simulink model "simulation_lab6"  (R2022b)
settings: Solver=FixedStepAuto  StartTime=0.0  StopTime=30  FixedStep=0.001  RelTol=1e-3
values from neighbouring files (symbols this model uses):
  A = double(subs(A,par,value))    [Lab6.m]    (also in Lab6_shu.m = [0  1                                                       )
  B = double(subs(B,par,value))    [Lab6.m]    (also in Lab6_shu.m = [0)
  C = [1 0 0 0;0 0 1 0]    [Lab6.m]    (also in Lab6_shu.m = [C1; C2])
  Cy = [1 0 0 0]    [Lab6.m]    (also in Lab6_shu.m)
  Cy_theta = [1 0 0 0;0 0 1 0]    [Lab6.m]    (also in Lab6_shu.m = [1 0 0 0; 0 0 1 0])
  D = zeros(2,1)    [Lab6.m]    (also in Lab6_shu.m = [0])
  Ly_fast = place(A',180/pi*Cy',poles_modified*6)'    [Lab6.m]    (also in Lab6_shu.m = (place(A',180/pi*Cy',6*poles))')
  Ly_slow = place(A',180/pi*Cy',poles_modified*3)'    [Lab6.m]    (also in Lab6_shu.m = (place(A',180/pi*Cy',3*poles))')
  Ly_theta_fast = place(A',180/pi*Cy_theta',poles_modified*6)'    [Lab6.m]    (also in Lab6_shu.m = (place(A',180/pi*Cy_theta',6*poles))')
  Ly_theta_slow = place(A',180/pi*Cy_theta',poles_modified*3)'    [Lab6.m]    (also in Lab6_shu.m = (place(A',180/pi*Cy_theta',3*poles))')
settings Model: Creator=me-clab2  LastModifiedBy=X1
settings SolverCC: AlgebraicLoopSolver=TrustRegion
settings DebuggingCC: UnconnectedInputMsg=warning  UnconnectedOutputMsg=warning  UnconnectedLineMsg=warning  SFMachineParentedDataDiag=warning
settings ModelReferenceCC: EnableRefExpFcnMdlSchedulingChecks=on

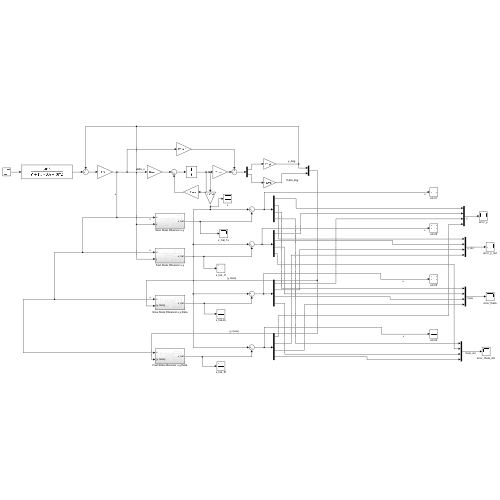
[thumbnail: Simulink's stored preview of the top-level diagram]
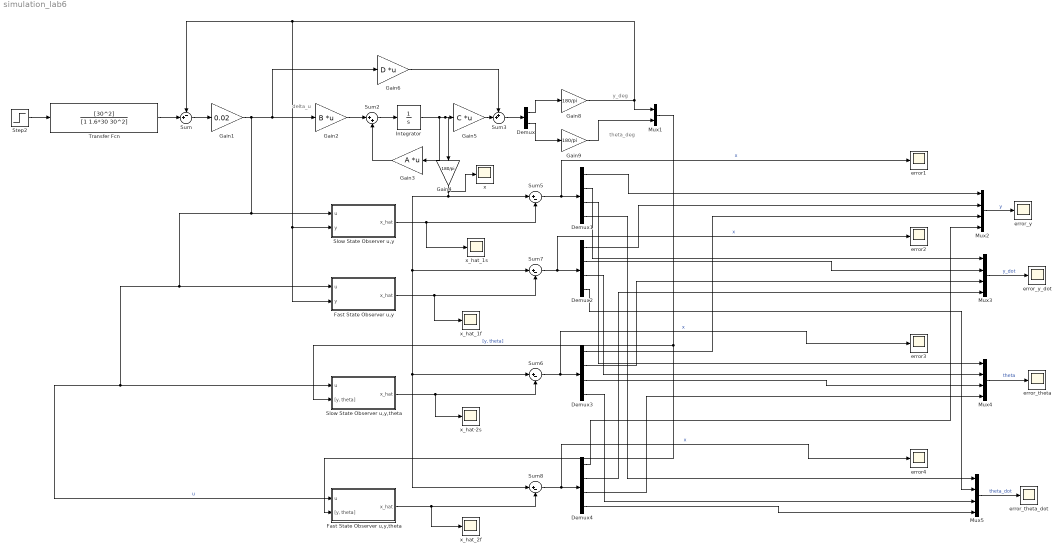
== system simulation_lab6 ==
  note: theta_deg
  note: y_deg
  note: delta_u
  Demux : Demux  Outputs=2
  Demux{1..4} (4 alike) : Demux
  Fast State Observer u,y : Subsystem
  Fast State Observer u,y,theta : Subsystem
  Gain1 : Gain  Gain=0.02
  Gain2 : Gain  Gain=B  Multiplication=Matrix(K*u) (u vector)
  Gain3 : Gain  Gain=A  Multiplication=Matrix(K*u) (u vector)
  Gain4 : Gain  Gain=180/pi
  Gain5 : Gain  Gain=C  Multiplication=Matrix(K*u) (u vector)
  Gain6 : Gain  Gain=D  Multiplication=Matrix(K*u) (u vector)
  Gain8 : Gain  Gain=180/pi
  Gain9 : Gain  Gain=180/pi
  Integrator : Integrator  InitialCondition=[0.01;0;0;0]
  Mux1 : Mux  Inputs=2
  Mux{2..5} (4 alike) : Mux
  "Slow State Observer u,y " : Subsystem
  Slow State Observer u,y,theta : Subsystem
  Step2 : Step  Time=0  After=30  SampleTime=0.001
  Sum : Sum  Inputs=-+|
  Sum2 : Sum  Inputs=|++
  Sum3 : Sum  Inputs=++|
  Sum{5..8} (4 alike) : Sum  Inputs=|+-
  Transfer Fcn : TransferFcn  Numerator=[30^2]  Denominator=[1 1.6*30 30^2]
  error{1..4} (4 alike) : Scope
  error_theta : Scope
  error_theta_dot : Scope
  error_y : Scope
  error_y_dot : Scope
  x : Scope
  x_hat-2s : Scope
  x_hat_1f : Scope
  x_hat_1s : Scope
  x_hat_2f : Scope
  wires:
  Sum2/1 -> Integrator/1
  Gain5/1 -> Sum3/2
  Sum/1 -> Gain1/1
  Gain6/1 -> Sum3/1
  Sum3/1 -> Demux/1
  Demux/1 -> Gain8/1
  Step2/1 -> Transfer Fcn/1
  Demux/2 -> Gain9/1
  Gain2/1 -> Sum2/1
  Gain3/1 -> Sum2/2
  Slow State Observer u,y,theta/1(x_hat) -> Sum6/2, x_hat-2s/1
  Gain9/1 -> Mux1/2
  Gain8/1 -> Fast State Observer u,y/2(y), "Slow State Observer u,y "/2(y), Sum/1, Mux1/1
  Fast State Observer u,y/1(x_hat) -> x_hat_1f/1, Sum7/2
  Integrator/1 -> Gain3/1, Gain5/1, Gain4/1
  Mux1/1 -> Fast State Observer u,y,theta/2("[y, theta]"), Slow State Observer u,y,theta/2("[y, theta]")  "[y, theta]"
  Fast State Observer u,y,theta/1(x_hat) -> Sum8/2, x_hat_2f/1
  Gain1/1 -> Gain2/1, Gain6/1, "Slow State Observer u,y "/1(u), Fast State Observer u,y/1(u), Slow State Observer u,y,theta/1(u), Fast State Observer u,y,theta/1(u)  "u"
  Demux1/1 -> Mux2/1
  Demux2/1 -> Mux2/2
  Demux3/1 -> Mux2/3
  Demux4/1 -> Mux2/4
  Demux3/2 -> Mux3/3
  Demux4/2 -> Mux3/4
  Demux2/2 -> Mux3/2
  Mux3/1 -> error_y_dot/1  "y_dot"
  Demux1/2 -> Mux3/1
  Demux3/3 -> Mux4/3
  Mux4/1 -> error_theta/1  "theta"
  Demux4/3 -> Mux4/4
  Demux2/3 -> Mux4/2
  Demux1/3 -> Mux4/1
  Demux3/4 -> Mux5/3
  Demux1/4 -> Mux5/1
  Demux4/4 -> Mux5/4
  Mux5/1 -> error_theta_dot/1  "theta_dot"
  Demux2/4 -> Mux5/2
  Transfer Fcn/1 -> Sum/2
  Gain4/1 -> Sum8/1, Sum6/1, Sum7/1, Sum5/1, x/1
  "Slow State Observer u,y "/1(x_hat) -> x_hat_1s/1, Sum5/2
  Sum8/1 -> error4/1, Demux4/1  "x"
  Sum6/1 -> error3/1, Demux3/1  "x"
  Sum5/1 -> error1/1, Demux1/1  "x"
  Sum7/1 -> error2/1, Demux2/1  "x"
  Mux2/1 -> error_y/1  "y"

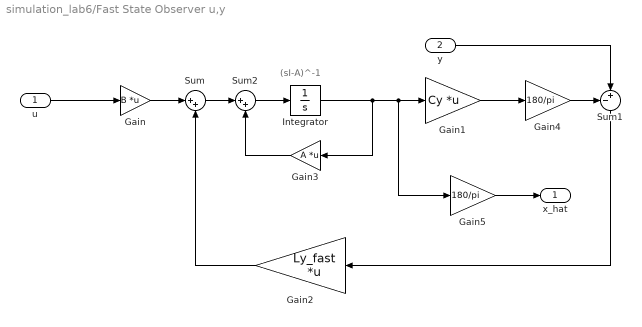
== system simulation_lab6/Fast State Observer u,y ==
  note: (sI-A)^-1
  u : Inport
  y : Inport  Port=2
  Gain : Gain  Gain=B  Multiplication=Matrix(K*u)
  Gain1 : Gain  Gain=Cy  Multiplication=Matrix(K*u)
  Gain2 : Gain  Gain=Ly_fast  Multiplication=Matrix(K*u)
  Gain3 : Gain  Gain=A  Multiplication=Matrix(K*u)
  Gain4 : Gain  Gain=180/pi
  Gain5 : Gain  Gain=180/pi
  Integrator : Integrator
  Sum : Sum  Inputs=|++
  Sum1 : Sum  Inputs=-+|
  Sum2 : Sum  Inputs=|++
  x_hat : Outport  VectorParamsAs1DForOutWhenUnconnected=off
  wires:
  u/1 -> Gain/1
  Gain/1 -> Sum/1
  Integrator/1 -> Gain3/1, Gain5/1, Gain1/1
  Gain1/1 -> Gain4/1
  y/1 -> Sum1/2
  Sum1/1 -> Gain2/1
  Gain2/1 -> Sum/2
  Sum/1 -> Sum2/1
  Sum2/1 -> Integrator/1
  Gain3/1 -> Sum2/2
  Gain4/1 -> Sum1/1
  Gain5/1 -> x_hat/1

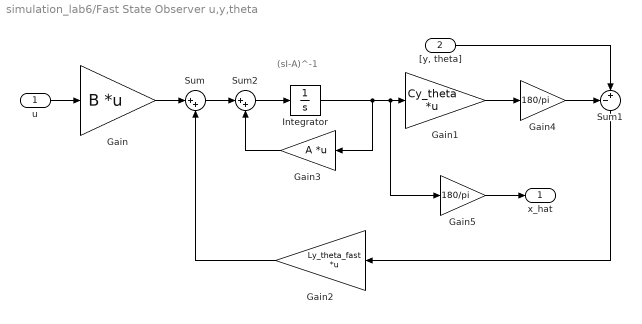
== system simulation_lab6/Fast State Observer u,y,theta ==
  note: (sI-A)^-1
  u : Inport
  "[y, theta]" : Inport  Port=2
  Gain : Gain  Gain=B  Multiplication=Matrix(K*u)
  Gain1 : Gain  Gain=Cy_theta  Multiplication=Matrix(K*u)
  Gain2 : Gain  Gain=Ly_theta_fast  Multiplication=Matrix(K*u)
  Gain3 : Gain  Gain=A  Multiplication=Matrix(K*u)
  Gain4 : Gain  Gain=180/pi
  Gain5 : Gain  Gain=180/pi
  Integrator : Integrator
  Sum : Sum  Inputs=|++
  Sum1 : Sum  Inputs=-+|
  Sum2 : Sum  Inputs=|++
  x_hat : Outport  VectorParamsAs1DForOutWhenUnconnected=off
  wires:
  u/1 -> Gain/1
  Gain/1 -> Sum/1
  Integrator/1 -> Gain3/1, Gain5/1, Gain1/1
  Gain1/1 -> Gain4/1
  "[y, theta]"/1 -> Sum1/2
  Sum1/1 -> Gain2/1
  Gain2/1 -> Sum/2
  Sum/1 -> Sum2/1
  Sum2/1 -> Integrator/1
  Gain3/1 -> Sum2/2
  Gain4/1 -> Sum1/1
  Gain5/1 -> x_hat/1

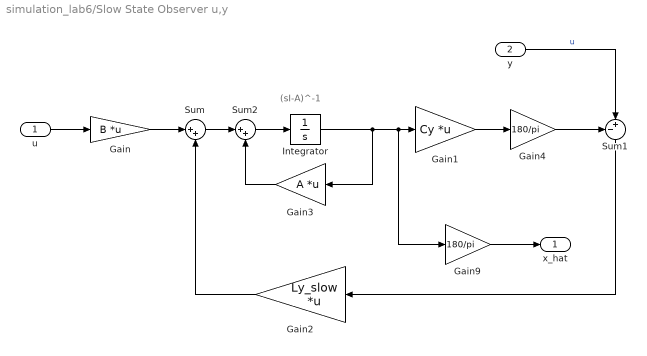
== system simulation_lab6/Slow State Observer u,y  ==
  note: (sI-A)^-1
  u : Inport
  y : Inport  Port=2
  Gain : Gain  Gain=B  Multiplication=Matrix(K*u) (u vector)
  Gain1 : Gain  Gain=Cy  Multiplication=Matrix(K*u) (u vector)
  Gain2 : Gain  Gain=Ly_slow  Multiplication=Matrix(K*u) (u vector)
  Gain3 : Gain  Gain=A  Multiplication=Matrix(K*u) (u vector)
  Gain4 : Gain  Gain=180/pi
  Gain9 : Gain  Gain=180/pi
  Integrator : Integrator
  Sum : Sum  Inputs=|++
  Sum1 : Sum  Inputs=-+|
  Sum2 : Sum  Inputs=|++
  x_hat : Outport  VectorParamsAs1DForOutWhenUnconnected=off
  wires:
  u/1 -> Gain/1
  Gain/1 -> Sum/1
  Integrator/1 -> Gain3/1, Gain9/1, Gain1/1
  Gain1/1 -> Gain4/1
  Sum1/1 -> Gain2/1
  Gain2/1 -> Sum/2
  Sum/1 -> Sum2/1
  Sum2/1 -> Integrator/1
  Gain3/1 -> Sum2/2
  y/1 -> Sum1/2  "u"
  Gain9/1 -> x_hat/1
  Gain4/1 -> Sum1/1

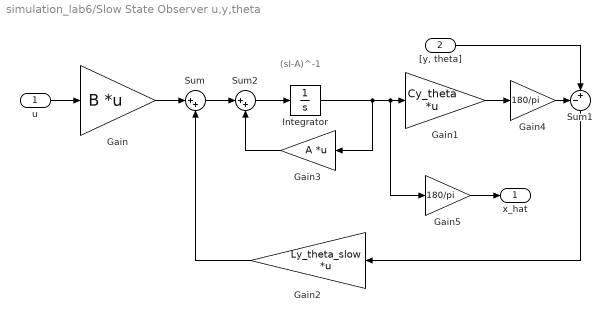
== system simulation_lab6/Slow State Observer u,y,theta ==
  note: (sI-A)^-1
  u : Inport
  "[y, theta]" : Inport  Port=2
  Gain : Gain  Gain=B  Multiplication=Matrix(K*u) (u vector)
  Gain1 : Gain  Gain=Cy_theta  Multiplication=Matrix(K*u) (u vector)
  Gain2 : Gain  Gain=Ly_theta_slow  Multiplication=Matrix(K*u) (u vector)
  Gain3 : Gain  Gain=A  Multiplication=Matrix(K*u) (u vector)
  Gain4 : Gain  Gain=180/pi
  Gain5 : Gain  Gain=180/pi
  Integrator : Integrator
  Sum : Sum  Inputs=|++
  Sum1 : Sum  Inputs=-+|
  Sum2 : Sum  Inputs=|++
  x_hat : Outport  VectorParamsAs1DForOutWhenUnconnected=off
  wires:
  u/1 -> Gain/1
  Gain/1 -> Sum/1
  Integrator/1 -> Gain3/1, Gain5/1, Gain1/1
  "[y, theta]"/1 -> Sum1/2
  Sum1/1 -> Gain2/1
  Gain2/1 -> Sum/2
  Sum/1 -> Sum2/1
  Sum2/1 -> Integrator/1
  Gain3/1 -> Sum2/2
  Gain1/1 -> Gain4/1
  Gain4/1 -> Sum1/1
  Gain5/1 -> x_hat/1
